simulink model "Trigonometry"  (R2020a)
settings: Solver=VariableStepAuto  StartTime=0.0  StopTime=10.0  RelTol=1e-3
settings Model: Creator=royde  LastModifiedBy=royde

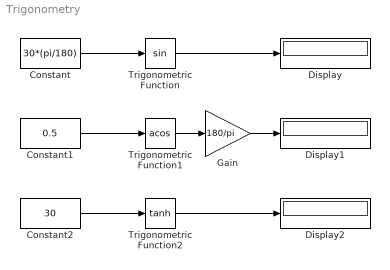
== system Trigonometry ==
  Constant : Constant  Value=30*(pi/180)
  Constant1 : Constant  Value=0.5
  Constant2 : Constant  Value=30
  Display : Display
  Display1 : Display
  Display2 : Display
  Gain : Gain  Gain=180/pi
  Trigonometric Function : Trigonometry
  Trigonometric Function1 : Trigonometry  Operator=acos
  Trigonometric Function2 : Trigonometry  Operator=tanh
  wires:
  Constant/1 -> Trigonometric Function/1
  Trigonometric Function/1 -> Display/1
  Trigonometric Function1/1 -> Gain/1
  Constant1/1 -> Trigonometric Function1/1
  Constant2/1 -> Trigonometric Function2/1
  Trigonometric Function2/1 -> Display2/1
  Gain/1 -> Display1/1
